simulink library "power_meter_iec"  (R2026a)
settings: Solver=VariableStepAuto
undefined symbols (not defined in the file): magnitude
libraries: $bdroot x11, moving_average_filter x1
settings Model: Creator=dbagn  LastModifiedBy=dbagn

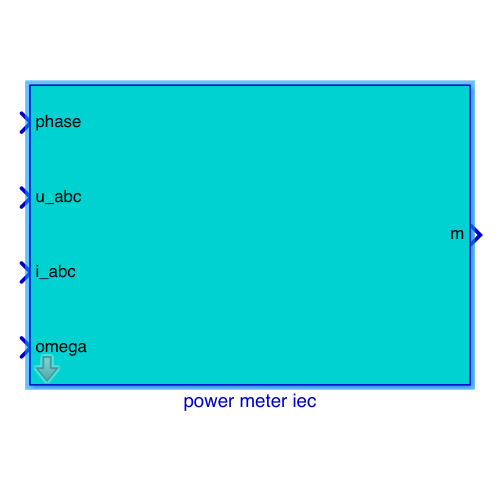
[thumbnail: Simulink's stored preview of the top-level diagram]
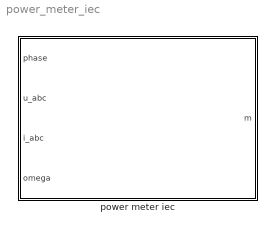
== system power_meter_iec ==
  power meter iec : Subsystem  mask{period=10e-3, ts=125e-6, enable_time=0.025}
      mask prompts: period "period (s)"; ts "sampling time (s)"; enable_time "enable_time (s)"

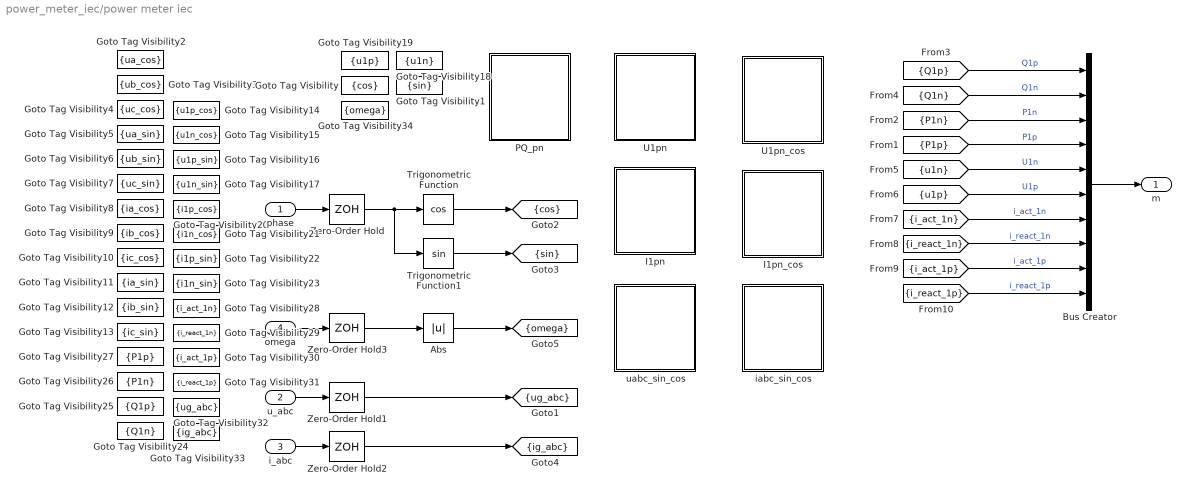
== system power_meter_iec/power meter iec ==
  phase : Inport
  u_abc : Inport  Port=2
  i_abc : Inport  Port=3
  omega : Inport  Port=4
  Abs : Abs  SaturateOnIntegerOverflow=off
  Bus Creator : BusCreator  Inputs=10
  Goto Tag Visibility : GotoTagVisibility  GotoTag=cos
  Goto Tag Visibility1 : GotoTagVisibility  GotoTag=sin
  Goto Tag Visibility10 : GotoTagVisibility  GotoTag=ic_cos
  Goto Tag Visibility11 : GotoTagVisibility  GotoTag=ia_sin
  Goto Tag Visibility12 : GotoTagVisibility  GotoTag=ib_sin
  Goto Tag Visibility13 : GotoTagVisibility  GotoTag=ic_sin
  Goto Tag Visibility14 : GotoTagVisibility  GotoTag=u1p_cos
  Goto Tag Visibility15 : GotoTagVisibility  GotoTag=u1n_cos
  Goto Tag Visibility16 : GotoTagVisibility  GotoTag=u1p_sin
  Goto Tag Visibility17 : GotoTagVisibility  GotoTag=u1n_sin
  Goto Tag Visibility18 : GotoTagVisibility  GotoTag=u1n
  Goto Tag Visibility19 : GotoTagVisibility  GotoTag=u1p
  Goto Tag Visibility2 : GotoTagVisibility  GotoTag=ua_cos
  Goto Tag Visibility20 : GotoTagVisibility  GotoTag=i1p_cos
  Goto Tag Visibility21 : GotoTagVisibility  GotoTag=i1n_cos
  Goto Tag Visibility22 : GotoTagVisibility  GotoTag=i1p_sin
  Goto Tag Visibility23 : GotoTagVisibility  GotoTag=i1n_sin
  Goto Tag Visibility24 : GotoTagVisibility  GotoTag=Q1n
  Goto Tag Visibility25 : GotoTagVisibility  GotoTag=Q1p
  Goto Tag Visibility26 : GotoTagVisibility  GotoTag=P1n
  Goto Tag Visibility27 : GotoTagVisibility  GotoTag=P1p
  Goto Tag Visibility28 : GotoTagVisibility  GotoTag=i_act_1n
  Goto Tag Visibility29 : GotoTagVisibility  GotoTag=i_react_1n
  Goto Tag Visibility3 : GotoTagVisibility  GotoTag=ub_cos
  Goto Tag Visibility30 : GotoTagVisibility  GotoTag=i_act_1p
  Goto Tag Visibility31 : GotoTagVisibility  GotoTag=i_react_1p
  Goto Tag Visibility32 : GotoTagVisibility  GotoTag=ug_abc
  Goto Tag Visibility33 : GotoTagVisibility  GotoTag=ig_abc
  Goto Tag Visibility34 : GotoTagVisibility  GotoTag=omega
  Goto Tag Visibility4 : GotoTagVisibility  GotoTag=uc_cos
  Goto Tag Visibility5 : GotoTagVisibility  GotoTag=ua_sin
  Goto Tag Visibility6 : GotoTagVisibility  GotoTag=ub_sin
  Goto Tag Visibility7 : GotoTagVisibility  GotoTag=uc_sin
  Goto Tag Visibility8 : GotoTagVisibility  GotoTag=ia_cos
  Goto Tag Visibility9 : GotoTagVisibility  GotoTag=ib_cos
  I1pn : Subsystem
  I1pn_cos : Subsystem
  PQ_pn : Subsystem
  Trigonometric Function : Trigonometry  Operator=cos
  Trigonometric Function1 : Trigonometry
  U1pn : Subsystem
  U1pn_cos : Subsystem
  Zero-Order Hold{,1..3} (4 alike) : ZeroOrderHold  SampleTime=ts
  iabc_sin_cos : Subsystem
  uabc_sin_cos : Subsystem
  m : Outport
  tag scope: cos=scoped, ig_abc=scoped, omega=scoped, sin=scoped, ug_abc=scoped
  wires:
  Trigonometric Function1/1 -> [sin]
  Trigonometric Function/1 -> [cos]
  phase/1 -> Zero-Order Hold/1
  [u1n] -> Bus Creator/5  "U1n"
  [u1p] -> Bus Creator/6  "U1p"
  [i_act_1n] -> Bus Creator/7  "i_act_1n"
  [i_react_1n] -> Bus Creator/8  "i_react_1n"
  [i_act_1p] -> Bus Creator/9  "i_act_1p"
  [i_react_1p] -> Bus Creator/10  "i_react_1p"
  u_abc/1 -> Zero-Order Hold1/1
  i_abc/1 -> Zero-Order Hold2/1
  Bus Creator/1 -> m/1
  Zero-Order Hold/1 -> Trigonometric Function/1, Trigonometric Function1/1
  Zero-Order Hold2/1 -> [ig_abc]
  Zero-Order Hold1/1 -> [ug_abc]
  omega/1 -> Zero-Order Hold3/1
  Zero-Order Hold3/1 -> Abs/1
  [P1p] -> Bus Creator/4  "P1p"
  [P1n] -> Bus Creator/3  "P1n"
  [Q1n] -> Bus Creator/2  "Q1n"
  [Q1p] -> Bus Creator/1  "Q1p"
  Abs/1 -> [omega]

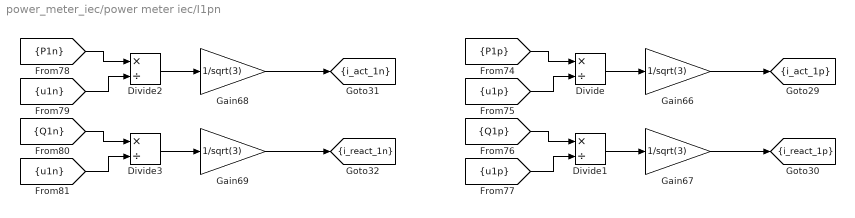
== system power_meter_iec/power meter iec/I1pn ==
  Divide{,1..3} (4 alike) : Product  Inputs=*/
  Gain{66..69} (4 alike) : Gain  Gain=1/sqrt(3)
  tag scope: i_act_1n=scoped, i_act_1p=scoped, i_react_1n=scoped, i_react_1p=scoped
  wires:
  [P1p] -> Divide/1
  Divide2/1 -> Gain68/1
  Gain68/1 -> [i_act_1n]
  [u1p] -> Divide1/2
  Gain67/1 -> [i_react_1p]
  [u1n] -> Divide2/2
  Gain66/1 -> [i_act_1p]
  Divide1/1 -> Gain67/1
  Divide3/1 -> Gain69/1
  Divide/1 -> Gain66/1
  [u1p] -> Divide/2
  Gain69/1 -> [i_react_1n]
  [Q1p] -> Divide1/1
  [u1n] -> Divide3/2
  [Q1n] -> Divide3/1
  [P1n] -> Divide2/1

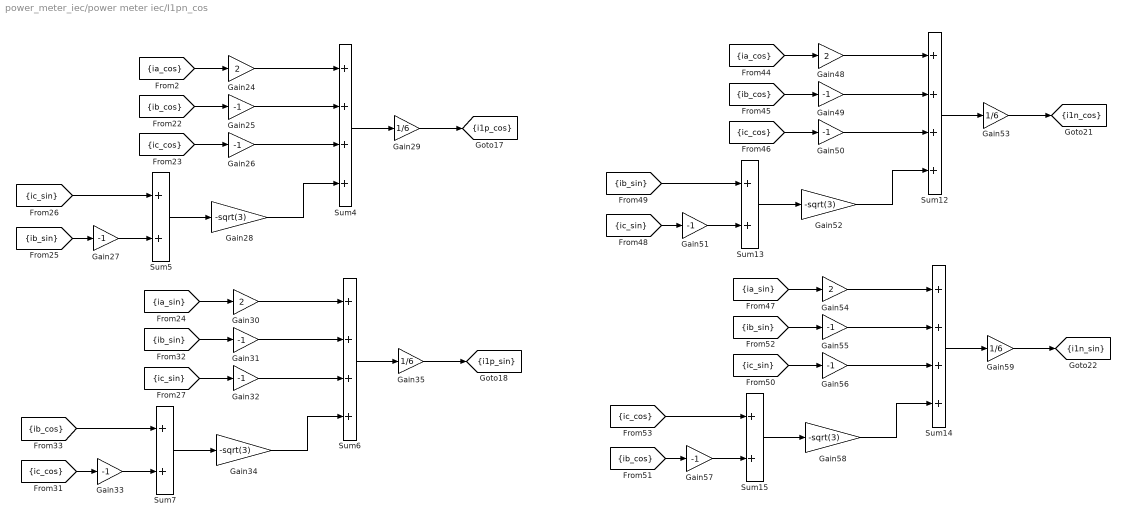
== system power_meter_iec/power meter iec/I1pn_cos ==
  Gain{24,30,48,54} (4 alike) : Gain  Gain=2
  Gain{25..27,31..33,49..51,55..57} (12 alike) : Gain  Gain=-1
  Gain{28,34,52,58} (4 alike) : Gain  Gain=-sqrt(3)
  Gain{29,35,53,59} (4 alike) : Gain  Gain=1/6
  Sum{4,6,12,14} (4 alike) : Sum  Inputs=++++
  Sum{5,7,13,15} (4 alike) : Sum
  tag scope: i1n_cos=scoped, i1n_sin=scoped, i1p_cos=scoped, i1p_sin=scoped
  wires:
  Gain35/1 -> [i1p_sin]
  Sum12/1 -> Gain53/1
  Gain27/1 -> Sum5/2
  Gain49/1 -> Sum12/2
  Gain54/1 -> Sum14/1
  [ib_cos] -> Sum7/1
  Gain52/1 -> Sum12/4
  Gain31/1 -> Sum6/2
  Sum14/1 -> Gain59/1
  [ic_sin] -> Gain51/1
  Gain29/1 -> [i1p_cos]
  [ic_sin] -> Gain32/1
  [ic_cos] -> Gain33/1
  Gain55/1 -> Sum14/2
  [ic_sin] -> Sum5/1
  Gain30/1 -> Sum6/1
  [ic_cos] -> Gain26/1
  [ia_cos] -> Gain48/1
  [ia_sin] -> Gain54/1
  Sum13/1 -> Gain52/1
  Sum4/1 -> Gain29/1
  Gain24/1 -> Sum4/1
  [ib_cos] -> Gain49/1
  [ib_sin] -> Sum13/1
  [ic_sin] -> Gain56/1
  Gain25/1 -> Sum4/2
  [ib_sin] -> Gain27/1
  Gain53/1 -> [i1n_cos]
  Sum7/1 -> Gain34/1
  Sum5/1 -> Gain28/1
  Gain33/1 -> Sum7/2
  [ib_cos] -> Gain57/1
  [ic_cos] -> Sum15/1
  Gain34/1 -> Sum6/4
  [ia_cos] -> Gain24/1
  Gain28/1 -> Sum4/4
  Gain32/1 -> Sum6/3
  [ib_sin] -> Gain55/1
  Gain26/1 -> Sum4/3
  Gain58/1 -> Sum14/4
  Gain59/1 -> [i1n_sin]
  Sum6/1 -> Gain35/1
  Gain51/1 -> Sum13/2
  [ia_sin] -> Gain30/1
  Gain48/1 -> Sum12/1
  [ic_cos] -> Gain50/1
  Gain56/1 -> Sum14/3
  [ib_sin] -> Gain31/1
  Gain50/1 -> Sum12/3
  Sum15/1 -> Gain58/1
  [ib_cos] -> Gain25/1
  Gain57/1 -> Sum15/2

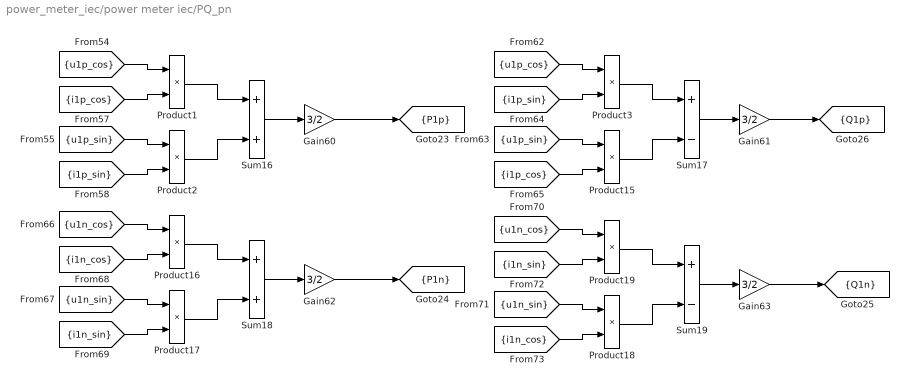
== system power_meter_iec/power meter iec/PQ_pn ==
  Gain{60..63} (4 alike) : Gain  Gain=3/2
  Product{1..3,15..19} (8 alike) : Product  RndMeth=Zero
  Sum16 : Sum
  Sum17 : Sum  Inputs=+-
  Sum18 : Sum
  Sum19 : Sum  Inputs=+-
  tag scope: P1n=scoped, P1p=scoped, Q1n=scoped, Q1p=scoped
  wires:
  [i1p_sin] -> Product2/2
  [i1n_sin] -> Product17/2
  Product19/1 -> Sum19/1
  Gain60/1 -> [P1p]
  Sum19/1 -> Gain63/1
  [u1n_cos] -> Product19/1
  [i1n_cos] -> Product16/2
  [i1n_cos] -> Product18/2
  Product16/1 -> Sum18/1
  Gain63/1 -> [Q1n]
  Product17/1 -> Sum18/2
  Product18/1 -> Sum19/2
  [u1p_cos] -> Product1/1
  Product1/1 -> Sum16/1
  Sum17/1 -> Gain61/1
  [i1p_cos] -> Product1/2
  Gain62/1 -> [P1n]
  Sum18/1 -> Gain62/1
  Gain61/1 -> [Q1p]
  Product2/1 -> Sum16/2
  [i1p_cos] -> Product15/2
  [u1p_sin] -> Product15/1
  Product15/1 -> Sum17/2
  [i1p_sin] -> Product3/2
  [u1p_sin] -> Product2/1
  [u1p_cos] -> Product3/1
  [u1n_sin] -> Product17/1
  [u1n_sin] -> Product18/1
  [u1n_cos] -> Product16/1
  Sum16/1 -> Gain60/1
  [i1n_sin] -> Product19/2
  Product3/1 -> Sum17/1

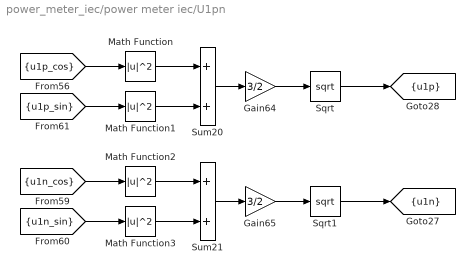
== system power_meter_iec/power meter iec/U1pn ==
  Gain64 : Gain  Gain=3/2
  Gain65 : Gain  Gain=3/2
  Math Function{,1..3} (4 alike) : Math  Operator=magnitude^2  SignedPower=on
  Sqrt : Sqrt
  Sqrt1 : Sqrt
  Sum20 : Sum
  Sum21 : Sum
  tag scope: u1n=scoped, u1p=scoped
  wires:
  Sum20/1 -> Gain64/1
  Math Function3/1 -> Sum21/2
  [u1p_cos] -> Math Function/1
  Math Function1/1 -> Sum20/2
  Math Function2/1 -> Sum21/1
  Sqrt1/1 -> [u1n]
  Gain64/1 -> Sqrt/1
  Sqrt/1 -> [u1p]
  Sum21/1 -> Gain65/1
  [u1n_sin] -> Math Function3/1
  Math Function/1 -> Sum20/1
  [u1n_cos] -> Math Function2/1
  Gain65/1 -> Sqrt1/1
  [u1p_sin] -> Math Function1/1

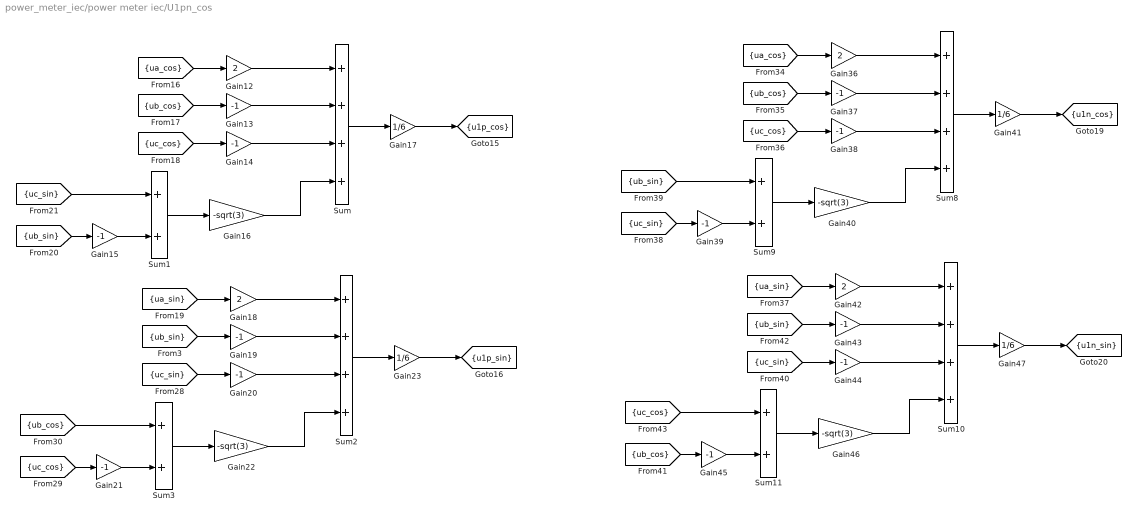
== system power_meter_iec/power meter iec/U1pn_cos ==
  Gain{12,18,36,42} (4 alike) : Gain  Gain=2
  Gain{13..15,19..21,37..39,43..45} (12 alike) : Gain  Gain=-1
  Gain{16,22,40,46} (4 alike) : Gain  Gain=-sqrt(3)
  Gain{17,23,41,47} (4 alike) : Gain  Gain=1/6
  Sum{,2,8,10} (4 alike) : Sum  Inputs=++++
  Sum{1,3,9,11} (4 alike) : Sum
  tag scope: u1n_cos=scoped, u1n_sin=scoped, u1p_cos=scoped, u1p_sin=scoped
  wires:
  Gain15/1 -> Sum1/2
  [ub_cos] -> Gain45/1
  [ub_cos] -> Gain37/1
  Gain13/1 -> Sum/2
  [ua_cos] -> Gain36/1
  Sum3/1 -> Gain22/1
  Gain40/1 -> Sum8/4
  Gain36/1 -> Sum8/1
  [ub_sin] -> Sum9/1
  Sum8/1 -> Gain41/1
  Sum11/1 -> Gain46/1
  [uc_sin] -> Gain20/1
  Gain39/1 -> Sum9/2
  [ua_cos] -> Gain12/1
  [ub_cos] -> Sum3/1
  [uc_sin] -> Gain44/1
  Gain42/1 -> Sum10/1
  Gain14/1 -> Sum/3
  Gain43/1 -> Sum10/2
  Sum/1 -> Gain17/1
  [uc_cos] -> Gain38/1
  Gain21/1 -> Sum3/2
  Gain41/1 -> [u1n_cos]
  Gain16/1 -> Sum/4
  [uc_sin] -> Sum1/1
  Gain37/1 -> Sum8/2
  Gain20/1 -> Sum2/3
  Gain44/1 -> Sum10/3
  [ub_cos] -> Gain13/1
  [ub_sin] -> Gain15/1
  [ub_sin] -> Gain43/1
  Sum1/1 -> Gain16/1
  [ua_sin] -> Gain42/1
  [uc_sin] -> Gain39/1
  Gain23/1 -> [u1p_sin]
  Gain38/1 -> Sum8/3
  [uc_cos] -> Gain14/1
  [uc_cos] -> Gain21/1
  Gain17/1 -> [u1p_cos]
  Sum10/1 -> Gain47/1
  Gain47/1 -> [u1n_sin]
  Gain46/1 -> Sum10/4
  Gain22/1 -> Sum2/4
  Gain19/1 -> Sum2/2
  Sum2/1 -> Gain23/1
  Gain45/1 -> Sum11/2
  [ub_sin] -> Gain19/1
  Gain18/1 -> Sum2/1
  [uc_cos] -> Sum11/1
  Sum9/1 -> Gain40/1
  [ua_sin] -> Gain18/1
  Gain12/1 -> Sum/1

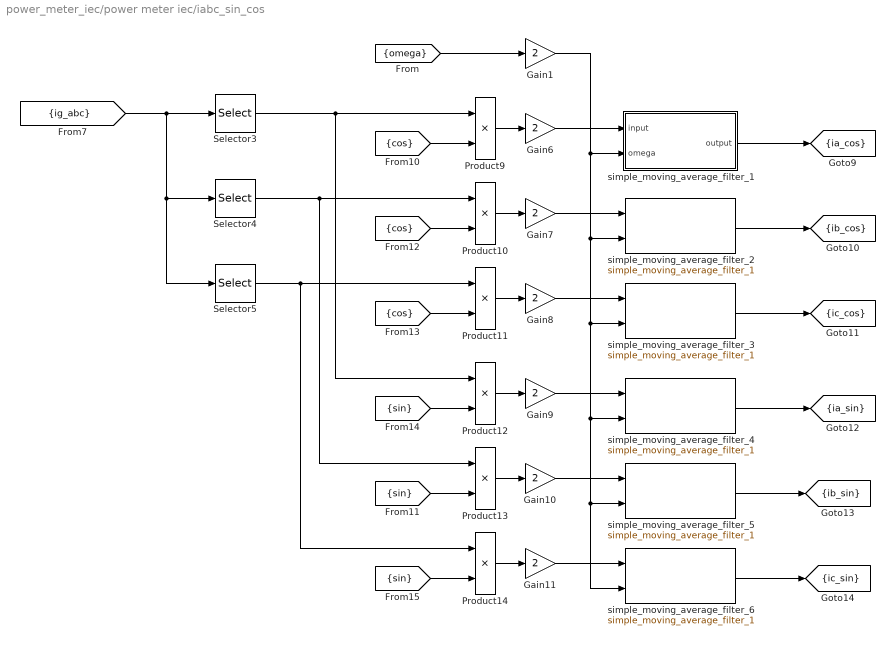
== system power_meter_iec/power meter iec/iabc_sin_cos ==
  Gain{1,6..11} (7 alike) : Gain  Gain=2
  Product{9..14} (6 alike) : Product  RndMeth=Zero
  Selector3 : Selector  InputPortWidth=3  IndexOptions=Index vector (dialog)  Indices=1  OutputSizes=1
  Selector4 : Selector  InputPortWidth=3  IndexOptions=Index vector (dialog)  Indices=2  OutputSizes=1
  Selector5 : Selector  InputPortWidth=3  IndexOptions=Index vector (dialog)  Indices=3  OutputSizes=1
  simple_moving_average_filter_1 : Subsystem
  simple_moving_average_filter_2 : $bdroot/power meter iec/iabc_sin_cos/simple_moving_average_filter_1  SystemSampleTime=-1  VariantActivationTime=update diagram  EmptyChoice=off  PassThrough=off  PassThroughVariantControl=(default)  EmptyChoiceVariantControl=(default)  AllowFlexibleInterface=on  Latency=0  AutoFrameSizeCalculation=off
      link override mavg_flt1: instance=1
  simple_moving_average_filter_3 : $bdroot/power meter iec/iabc_sin_cos/simple_moving_average_filter_1  SystemSampleTime=-1  VariantActivationTime=update diagram  EmptyChoice=off  PassThrough=off  PassThroughVariantControl=(default)  EmptyChoiceVariantControl=(default)  AllowFlexibleInterface=on  Latency=0  AutoFrameSizeCalculation=off
      link override mavg_flt1: instance=2
  simple_moving_average_filter_4 : $bdroot/power meter iec/iabc_sin_cos/simple_moving_average_filter_1  SystemSampleTime=-1  VariantActivationTime=update diagram  EmptyChoice=off  PassThrough=off  PassThroughVariantControl=(default)  EmptyChoiceVariantControl=(default)  AllowFlexibleInterface=on  Latency=0  AutoFrameSizeCalculation=off
      link override mavg_flt1: instance=3
  simple_moving_average_filter_5 : $bdroot/power meter iec/iabc_sin_cos/simple_moving_average_filter_1  SystemSampleTime=-1  VariantActivationTime=update diagram  EmptyChoice=off  PassThrough=off  PassThroughVariantControl=(default)  EmptyChoiceVariantControl=(default)  AllowFlexibleInterface=on  Latency=0  AutoFrameSizeCalculation=off
      link override mavg_flt1: instance=4
  simple_moving_average_filter_6 : $bdroot/power meter iec/iabc_sin_cos/simple_moving_average_filter_1  SystemSampleTime=-1  VariantActivationTime=update diagram  EmptyChoice=off  PassThrough=off  PassThroughVariantControl=(default)  EmptyChoiceVariantControl=(default)  AllowFlexibleInterface=on  Latency=0  AutoFrameSizeCalculation=off
      link override mavg_flt1: instance=5
  tag scope: ia_cos=scoped, ia_sin=scoped, ib_cos=scoped, ib_sin=scoped, ic_cos=scoped, ic_sin=scoped
  wires:
  Selector5/1 -> Product11/1, Product14/1
  Product13/1 -> Gain10/1
  Product12/1 -> Gain9/1
  Gain8/1 -> simple_moving_average_filter_3/1
  [cos] -> Product11/2
  [ig_abc] -> Selector3/1, Selector4/1, Selector5/1
  [sin] -> Product13/2
  Product11/1 -> Gain8/1
  Gain9/1 -> simple_moving_average_filter_4/1
  [cos] -> Product9/2
  [cos] -> Product10/2
  Gain7/1 -> simple_moving_average_filter_2/1
  Selector3/1 -> Product9/1, Product12/1
  Gain10/1 -> simple_moving_average_filter_5/1
  Product10/1 -> Gain7/1
  Product9/1 -> Gain6/1
  [sin] -> Product14/2
  Selector4/1 -> Product10/1, Product13/1
  Gain11/1 -> simple_moving_average_filter_6/1
  [sin] -> Product12/2
  Product14/1 -> Gain11/1
  simple_moving_average_filter_2/1 -> [ib_cos]
  simple_moving_average_filter_6/1 -> [ic_sin]
  simple_moving_average_filter_4/1 -> [ia_sin]
  simple_moving_average_filter_3/1 -> [ic_cos]
  simple_moving_average_filter_5/1 -> [ib_sin]
  Gain6/1 -> simple_moving_average_filter_1/1(input)
  simple_moving_average_filter_1/1(output) -> [ia_cos]
  [omega] -> Gain1/1
  Gain1/1 -> simple_moving_average_filter_2/2, simple_moving_average_filter_3/2, simple_moving_average_filter_4/2, simple_moving_average_filter_6/2, simple_moving_average_filter_5/2, simple_moving_average_filter_1/2(omega)

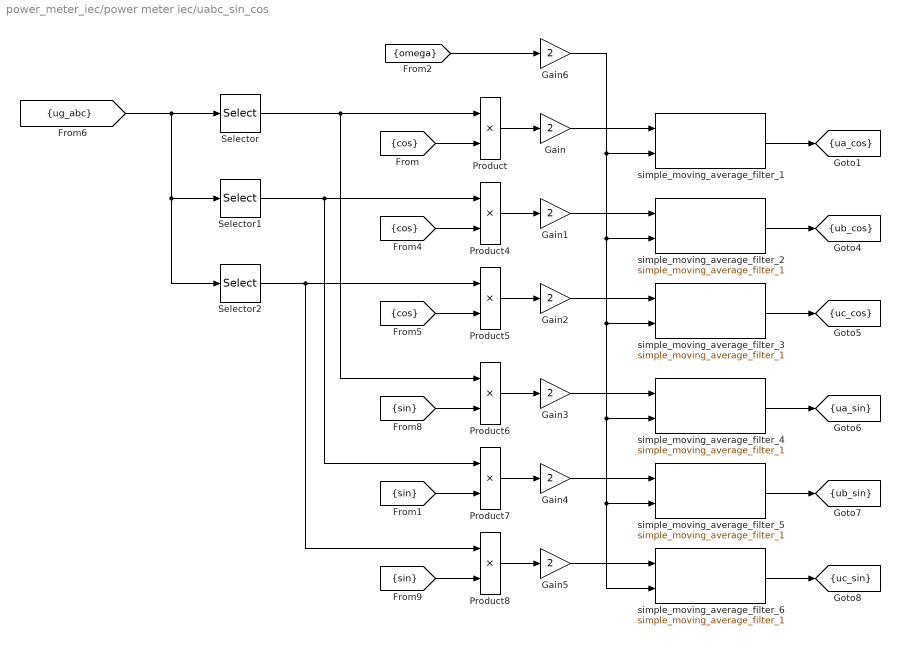
== system power_meter_iec/power meter iec/uabc_sin_cos ==
  Gain{,1..6} (7 alike) : Gain  Gain=2
  Product{,4..8} (6 alike) : Product  RndMeth=Zero
  Selector : Selector  InputPortWidth=3  IndexOptions=Index vector (dialog)  Indices=1  OutputSizes=1
  Selector1 : Selector  InputPortWidth=3  IndexOptions=Index vector (dialog)  Indices=2  OutputSizes=1
  Selector2 : Selector  InputPortWidth=3  IndexOptions=Index vector (dialog)  Indices=3  OutputSizes=1
  simple_moving_average_filter_1 : $bdroot/power meter iec/iabc_sin_cos/simple_moving_average_filter_1  SystemSampleTime=-1  VariantActivationTime=update diagram  EmptyChoice=off  PassThrough=off  PassThroughVariantControl=(default)  EmptyChoiceVariantControl=(default)  AllowFlexibleInterface=on  Latency=0  AutoFrameSizeCalculation=off
      link override mavg_flt1: instance=6
  simple_moving_average_filter_2 : $bdroot/power meter iec/iabc_sin_cos/simple_moving_average_filter_1  SystemSampleTime=-1  VariantActivationTime=update diagram  EmptyChoice=off  PassThrough=off  PassThroughVariantControl=(default)  EmptyChoiceVariantControl=(default)  AllowFlexibleInterface=on  Latency=0  AutoFrameSizeCalculation=off
      link override mavg_flt1: instance=7
  simple_moving_average_filter_3 : $bdroot/power meter iec/iabc_sin_cos/simple_moving_average_filter_1  SystemSampleTime=-1  VariantActivationTime=update diagram  EmptyChoice=off  PassThrough=off  PassThroughVariantControl=(default)  EmptyChoiceVariantControl=(default)  AllowFlexibleInterface=on  Latency=0  AutoFrameSizeCalculation=off
      link override mavg_flt1: instance=8
  simple_moving_average_filter_4 : $bdroot/power meter iec/iabc_sin_cos/simple_moving_average_filter_1  SystemSampleTime=-1  VariantActivationTime=update diagram  EmptyChoice=off  PassThrough=off  PassThroughVariantControl=(default)  EmptyChoiceVariantControl=(default)  AllowFlexibleInterface=on  Latency=0  AutoFrameSizeCalculation=off
      link override mavg_flt1: instance=9
  simple_moving_average_filter_5 : $bdroot/power meter iec/iabc_sin_cos/simple_moving_average_filter_1  SystemSampleTime=-1  VariantActivationTime=update diagram  EmptyChoice=off  PassThrough=off  PassThroughVariantControl=(default)  EmptyChoiceVariantControl=(default)  AllowFlexibleInterface=on  Latency=0  AutoFrameSizeCalculation=off
      link override mavg_flt1: instance=10
  simple_moving_average_filter_6 : $bdroot/power meter iec/iabc_sin_cos/simple_moving_average_filter_1  SystemSampleTime=-1  VariantActivationTime=update diagram  EmptyChoice=off  PassThrough=off  PassThroughVariantControl=(default)  EmptyChoiceVariantControl=(default)  AllowFlexibleInterface=on  Latency=0  AutoFrameSizeCalculation=off
      link override mavg_flt1: instance=11
  tag scope: ua_cos=scoped, ua_sin=scoped, ub_cos=scoped, ub_sin=scoped, uc_cos=scoped, uc_sin=scoped
  wires:
  Product/1 -> Gain/1
  Gain1/1 -> simple_moving_average_filter_2/1
  [cos] -> Product4/2
  Gain5/1 -> simple_moving_average_filter_6/1
  [ug_abc] -> Selector2/1, Selector1/1, Selector/1
  Product5/1 -> Gain2/1
  Gain3/1 -> simple_moving_average_filter_4/1
  Gain2/1 -> simple_moving_average_filter_3/1
  Gain/1 -> simple_moving_average_filter_1/1
  [sin] -> Product8/2
  Product4/1 -> Gain1/1
  Selector/1 -> Product6/1, Product/1
  Product7/1 -> Gain4/1
  Gain4/1 -> simple_moving_average_filter_5/1
  Selector1/1 -> Product7/1, Product4/1
  [sin] -> Product7/2
  Product6/1 -> Gain3/1
  [cos] -> Product5/2
  Product8/1 -> Gain5/1
  [sin] -> Product6/2
  [cos] -> Product/2
  Selector2/1 -> Product8/1, Product5/1
  simple_moving_average_filter_1/1 -> [ua_cos]
  simple_moving_average_filter_2/1 -> [ub_cos]
  simple_moving_average_filter_3/1 -> [uc_cos]
  simple_moving_average_filter_4/1 -> [ua_sin]
  simple_moving_average_filter_5/1 -> [ub_sin]
  simple_moving_average_filter_6/1 -> [uc_sin]
  Gain6/1 -> simple_moving_average_filter_1/2, simple_moving_average_filter_2/2, simple_moving_average_filter_3/2, simple_moving_average_filter_4/2, simple_moving_average_filter_5/2, simple_moving_average_filter_6/2
  [omega] -> Gain6/1

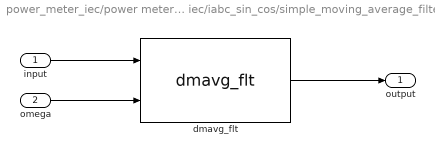
== system power_meter_iec/power meter iec/iabc_sin_cos/simple_moving_average_filter_1 ==
  input : Inport
  omega : Inport  Port=2
  dmavg_flt : moving_average_filter/dmavg_flt  ts=ts  enable_time=enable_time
  output : Outport
  wires:
  input/1 -> dmavg_flt/1
  omega/1 -> dmavg_flt/2
  dmavg_flt/1 -> output/1
